simulink model "QRotorSimulation"  (R2022a)
settings: Solver=VariableStepAuto  StartTime=0.0  StopTime=10.0  RelTol=1e-9
settings Model: Creator=carlossilvestre  LastModifiedBy=FLKU
settings SolverCC: AlgebraicLoopSolver=TrustRegion
settings DebuggingCC: UnconnectedInputMsg=warning  UnconnectedOutputMsg=warning  UnconnectedLineMsg=warning  SFMachineParentedDataDiag=warning

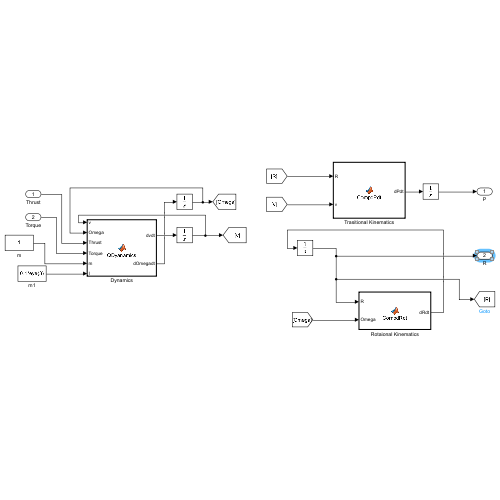
[thumbnail: Simulink's stored preview of the top-level diagram]
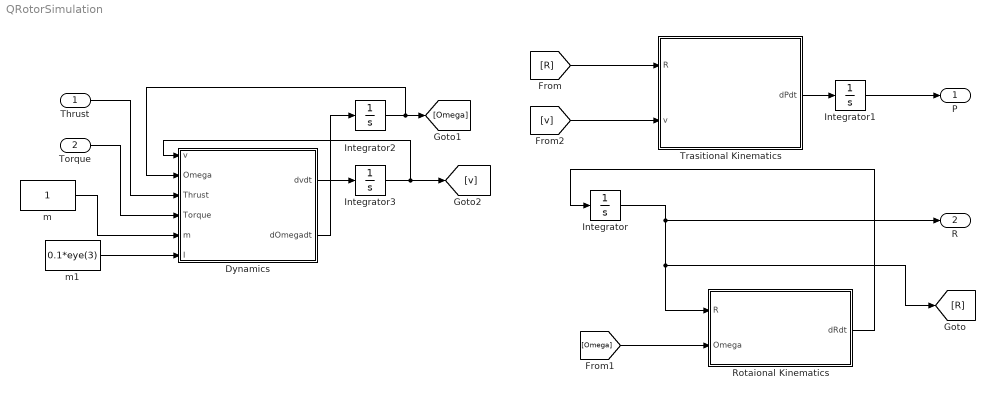
== system QRotorSimulation ==
  Thrust : Inport
  Torque : Inport  Port=2
  Dynamics : MATLAB Function  TreatAsAtomicUnit=on
  Integrator : Integrator  InitialCondition=eye(3)
  Integrator1 : Integrator  InitialCondition=[0,0,0]
  Integrator2 : Integrator  InitialCondition=[0,0,0]  ContinuousStateAttributes='omega'
  Integrator3 : Integrator  InitialCondition=[0,0,0]  ContinuousStateAttributes='velocity'
  Rotaional Kinematics : MATLAB Function  TreatAsAtomicUnit=on
  Trasitional Kinematics : MATLAB Function  TreatAsAtomicUnit=on
  m : Constant
  m1 : Constant  Value=0.1*eye(3)
  P : Outport
  R : Outport  Port=2
  wires:
  Dynamics/1(dvdt) -> Integrator3/1
  Integrator2/1 -> [Omega], Dynamics/2(Omega)
  Rotaional Kinematics/1(dRdt) -> Integrator/1
  Thrust/1 -> Dynamics/3(Thrust)
  Dynamics/2(dOmegadt) -> Integrator2/1
  m1/1 -> Dynamics/6(I)
  [R] -> Trasitional Kinematics/1(R)
  Trasitional Kinematics/1(dPdt) -> Integrator1/1
  Torque/1 -> Dynamics/4(Torque)
  [Omega] -> Rotaional Kinematics/2(Omega)
  [v] -> Trasitional Kinematics/2(v)
  m/1 -> Dynamics/5(m)
  Integrator/1 -> Rotaional Kinematics/1(R), [R], R/1
  Integrator3/1 -> [v], Dynamics/1(v)
  Integrator1/1 -> P/1

== matlab function QRotorSimulation/Trasitional Kinematics ==
  data: R input; dPdt output; v input
function dPdt = CompdPdt(R,v)
dPdt=R*v;
end

== matlab function QRotorSimulation/Rotaional Kinematics ==
  data: R input; dRdt output; Omega input
function dRdt = CompdRdt(R,Omega)
dRdt=R*skew(Omega);
end

== matlab function QRotorSimulation/Dynamics ==
  data: v input; Omega input; dvdt output; Thrust input; Torque input; dOmegadt output; m input; I input
function [dvdt,dOmegadt] = QDyanamics(v,Omega,Thrust,Torque,m,I)
m=0.1;
I=eye(3)*0.1;
dvdt=-skew(Omega)*v+1/m*Thrust;
dOmegadt=-I^-1*skew(Omega)*I*W+I^-1*Torque;
end
